simulink model "ekfPendulum"  (R2023a)
settings: Solver=VariableStepAuto  StartTime=0.0  StopTime=30  RelTol=1e-3
libraries: simulink x1, sharedTrackingLibrary x1
settings Model: Creator=idlsa  LastModifiedBy=idlsa

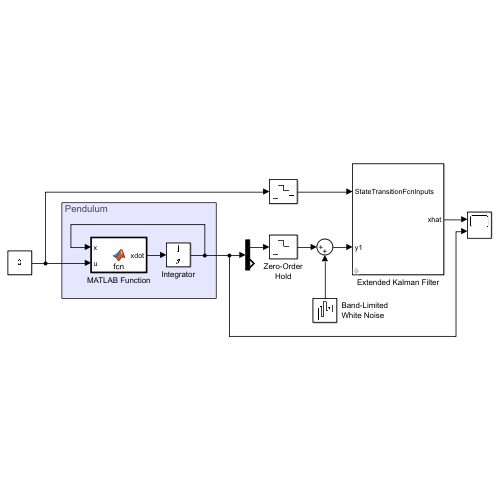
[thumbnail: Simulink's stored preview of the top-level diagram]
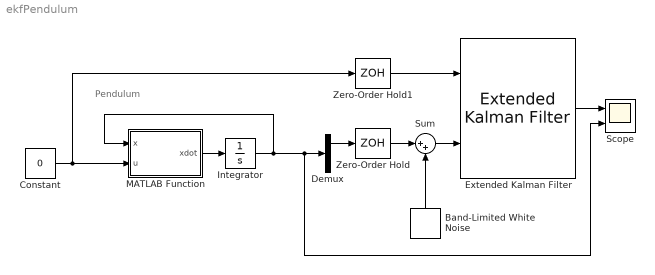
== system ekfPendulum ==
  note: Pendulum
  Band-Limited White Noise : simulink/Sources/Band-Limited White Noise  Cov=[0.01]*0.01  Ts=0.01  seed=[23341]
  Constant : Constant  Value=0
  Demux : Demux  Outputs=2
  Extended Kalman Filter : sharedTrackingLibrary/Extended Kalman Filter  StateTransitionFcn=funTran  HasStateTransitionJacobianFcn=off  HasAdditiveProcessNoise=Additive  ProcessNoise=diag([1e-5,1e-5])  HasTimeVaryingProcessNoise=off  HasStateTransitionFcnExtraArgument=1  InitialState=[0;0]  InitialStateCovariance=1  MeasurementFcn1=funMeas  HasMeasurementJacobianFcn1=off  HasMeasurementEnablePort1=off  HasAdditiveMeasurementNoise1=Additive  MeasurementNoise1=1e-2  HasTimeVaryingMeasurementNoise1=off  HasMeasurementFcnExtraArgument1=0  HasMeasurementWrapping1=off  MeasurementFcn2=myMeasurementFcn  HasMeasurementJacobianFcn2=off  HasMeasurementEnablePort2=off  HasAdditiveMeasurementNoise2=Additive  MeasurementNoise2=1  HasTimeVaryingMeasurementNoise2=off  HasMeasurementFcnExtraArgument2=0  HasMeasurementWrapping2=off  MeasurementFcn3=myMeasurementFcn  HasMeasurementJacobianFcn3=off  HasMeasurementEnablePort3=off  HasAdditiveMeasurementNoise3=Additive  MeasurementNoise3=1  HasTimeVaryingMeasurementNoise3=off  HasMeasurementFcnExtraArgument3=0  HasMeasurementWrapping3=off  MeasurementFcn4=myMeasurementFcn  HasMeasurementJacobianFcn4=off  HasMeasurementEnablePort4=off  HasAdditiveMeasurementNoise4=Additive  MeasurementNoise4=1  HasTimeVaryingMeasurementNoise4=off  HasMeasurementFcnExtraArgument4=0  HasMeasurementWrapping4=off  MeasurementFcn5=myMeasurementFcn  HasMeasurementJacobianFcn5=off  HasMeasurementEnablePort5=off  HasAdditiveMeasurementNoise5=Additive  MeasurementNoise5=1  HasTimeVaryingMeasurementNoise5=off  HasMeasurementFcnExtraArgument5=0  HasMeasurementWrapping5=off  EnableMultirate=off  StateTransitionFcnSampleTime=1  MeasurementFcn1SampleTime=1  MeasurementFcn2SampleTime=1  MeasurementFcn3SampleTime=1  MeasurementFcn4SampleTime=1  MeasurementFcn5SampleTime=1  UseCurrentEstimator=on  OutputStateCovariance=off  DataType=double  SampleTime=0.01  NumberOfMeasurements=1
  Integrator : Integrator  InitialCondition=[pi/4;0]
  MATLAB Function : MATLAB Function  TreatAsAtomicUnit=on
  Scope : Scope  NumInputPorts=2
  Sum : Sum  Inputs=|++
  Zero-Order Hold : ZeroOrderHold  SampleTime=0.01
  Zero-Order Hold1 : ZeroOrderHold  SampleTime=0.01
  wires:
  Integrator/1 -> Scope/2, Demux/1, MATLAB Function/1(x)
  Constant/1 -> Zero-Order Hold1/1, MATLAB Function/2(u)
  MATLAB Function/1(xdot) -> Integrator/1
  Demux/1 -> Zero-Order Hold/1
  Zero-Order Hold1/1 -> Extended Kalman Filter/1
  Extended Kalman Filter/1 -> Scope/1
  Zero-Order Hold/1 -> Sum/1
  Sum/1 -> Extended Kalman Filter/2
  Band-Limited White Noise/1 -> Sum/2

== matlab function ekfPendulum/MATLAB Function ==
  data: x input; u input; xdot output
function xdot = fcn(x,u)
m = 1; l = 0.5; g = 9.8;
xdot = [x(2);1/(m*l^2)*u-g/l*sin(x(1))];
